simulink model "xianxingfangzhen"  (R2018a)
settings: Solver=FixedStepAuto  StartTime=0.0  StopTime=10  FixedStep=0.01  RelTol=1e-3
values from neighbouring files (symbols this model uses):
  A_LAT = [Ybeita alpha+Yp Yr-1 g*cos(alpha)/V;Lbeita1 Lp1 Lr1 0;Nbeita1 Np1 Nr1 0;0 1 tan(alpha) 0]    [calculate.m]
  A_LON = [Xv Xa+g 0 -g;-Zv -Za 1 0;Mv-Ma1*Zv Ma-Ma1*Za Mq+Ma1 0;0 0 1 0]    [calculate.m]
  B_LAT = [0 Ydeltar;Ldeltaa1 Ldeltar1;Ndeltaa1 Ndeltar1;0 0]    [calculate.m]
  B_LON = [Xdeltae Xdeltap;-Zdeltae -Zdeltap;Mdeltae-Ma1*Zdeltae Mdeltap-Ma1*Zdeltap;0 0]    [calculate.m]
  C = [1 0 0 0;0 1 0 0;0 0 1 0;0 0 0 1]    [calculate.m]
  D = zeros(4,2)    [calculate.m]
  ini_state_LON = zeros(4,1)    [calculate.m]
settings Model: Creator=87138  LastModifiedBy=87138

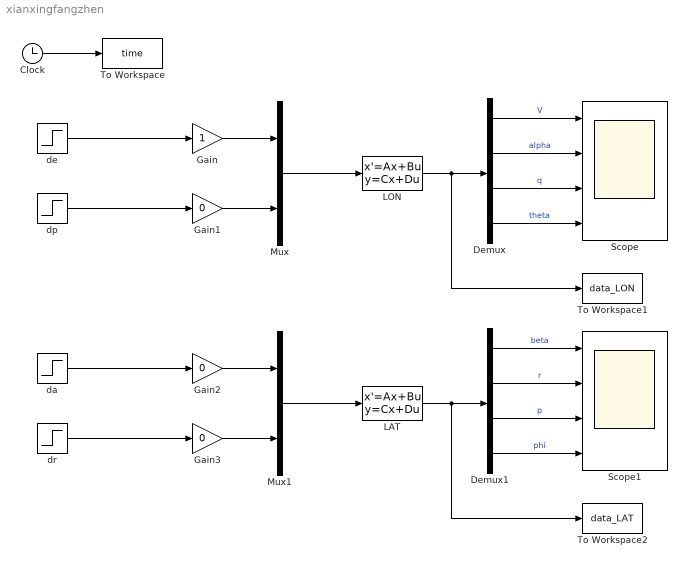
== system xianxingfangzhen ==
  Clock : Clock
  Demux : Demux
  Demux1 : Demux
  Gain : Gain
  Gain1 : Gain  Gain=0
  Gain2 : Gain  Gain=0
  Gain3 : Gain  Gain=0
  LAT : StateSpace  A=A_LAT  B=B_LAT  C=C  D=D  InitialCondition=ini_state_LON
  LON : StateSpace  A=A_LON  B=B_LON  C=C  D=D  InitialCondition=ini_state_LON
  Mux : Mux  Inputs=2
  Mux1 : Mux  Inputs=2
  Scope : Scope  NumInputPorts=4
  Scope1 : Scope  NumInputPorts=4
  To Workspace : ToWorkspace  VariableName=time  SampleTime=-1
      settings: Save2DSignal=2-D array (concatenate along first dimension)
  To Workspace1 : ToWorkspace  VariableName=data_LON  SampleTime=-1
      settings: Save2DSignal=2-D array (concatenate along first dimension)
  To Workspace2 : ToWorkspace  VariableName=data_LAT  SampleTime=-1
      settings: Save2DSignal=2-D array (concatenate along first dimension)
  da : Step  Time=0.01  SampleTime=0
  de : Step  Time=0.01  SampleTime=0
  dp : Step  Time=0.01  SampleTime=0
  dr : Step  Time=0.01  SampleTime=0
  wires:
  Clock/1 -> To Workspace/1
  Gain/1 -> Mux/1
  Gain1/1 -> Mux/2
  Mux/1 -> LON/1
  de/1 -> Gain/1
  dp/1 -> Gain1/1
  LON/1 -> To Workspace1/1, Demux/1
  Demux/1 -> Scope/1  "V"
  Demux/2 -> Scope/2  "alpha"
  Demux/3 -> Scope/3  "q"
  Demux/4 -> Scope/4  "theta"
  Demux1/4 -> Scope1/4  "phi"
  Demux1/2 -> Scope1/2  "r"
  Gain2/1 -> Mux1/1
  Mux1/1 -> LAT/1
  LAT/1 -> To Workspace2/1, Demux1/1
  Gain3/1 -> Mux1/2
  da/1 -> Gain2/1
  Demux1/3 -> Scope1/3  "p"
  dr/1 -> Gain3/1
  Demux1/1 -> Scope1/1  "beta"
